simulink model "HQEV_MiL_20160830_integrate_r2017a"  (Simulink 8.9)
settings: Solver=FixedStepDiscrete  StartTime=0.0  StopTime=inf  FixedStep=0.01  RelTol=1e-3  EnableMultiTasking=on
PostLoadFcn:
  | , if any(exist('dsrtsu_mdlpostloadfcn', 'file') == [2, 3, 6]), try dsrtsu_mdlpostloadfcn('Execute', bdroot); catch fprintf('Error in PostLoadFcn (dsrtsu_mdlpostloadfcn) for model "%s":\n %s\n', bdroot, lasterr); end, end,
values from neighbouring files (symbols this model uses):
  Bat_C_Ah = 36    [parameter_V1.mat]
  Bat_ocv_xIndex = [5 10 20 30 40 50 60 70 80 90 95]    [parameter_V1.mat]
  Bat_ocv_z = [329 332 340 345 347 351 358 372 377 386 391]    [parameter_V1.mat]
  Bat_R_ohm_z = [4.41 3.46 1.57 1.07 0.76 0.63 0.55 0.44 0.41 0.4 0.4 3.14 ... (66 elements, 11x6)]    [parameter_V1.mat]
  Bat_SOC_Init = 90    [parameter_V1.mat]
  Env_hum_pct_Ambient = 30    [parameter_V1.mat]
  Env_Slope_deg = 0    [parameter_V1.mat]
  Env_Temp_degC_Ambient = 25    [parameter_V1.mat]
  Env_v_kmph_HWind = 0    [parameter_V1.mat]
  Reducer_F_i = 7.23    [parameter_V1.mat]
  Reducer_R_i = 7.23    [parameter_V1.mat]
  Veh =     [parameter_V1.mat]
  Veh_A_m2_Fr = 2.246    [parameter_V1.mat]
  Veh_F_Brake =     [parameter_V1.mat]
  Veh_fac_AirDrag = 0.326    [parameter_V1.mat]
  Veh_fac_WhDragFrict_0 = 0.011    [parameter_V1.mat]
  Veh_g_mps2_C = 9.81    [parameter_V1.mat]
  Veh_GainBrake =     [parameter_V1.mat]
  Veh_h_m_COGHigh = 0.5    [parameter_V1.mat]
  Veh_J_kgm2_Wh = 1.3635    [parameter_V1.mat]
  Veh_L_m_AxlBas = 2.63    [parameter_V1.mat]
  Veh_M_kg = 1427    [parameter_V1.mat]
  Veh_mu_Brake = 0.4    [parameter_V1.mat]
  Veh_mu_Tyre =     [parameter_V1.mat]
  Veh_num_FrictPair = 8    [parameter_V1.mat]
  Veh_pct_Brk = 70    [parameter_V1.mat]
  Veh_r_dyn =     [parameter_V1.mat]
  Veh_r_m_BrkDisk = 0.136    [parameter_V1.mat]
  Veh_rho_kgpm3_Air = 1.2258    [parameter_V1.mat]
undefined symbols (not defined in the file or in its folder): DiscIntNeverNeededParam, p_bool_False_M, p_bool_True_M
libraries: BaseOperationLib_Browser x38, simulink x8, DTQC_lib x1, ERR_lib x1, MQM_lib x1, PTCL_lib x1, PUD_lib x1, TQD_lib x1, TQR_lib x1, VMM_lib x1, ACCA_lib x1, BBCA_lib x1
(part 9 of 15)

== system HQEV_MiL_20160830_integrate_r2017a/MiL/Test_Integration/MCU_RR/MCU/Signal/MCU2_TMSpeed ==
  In1 : Inport
  Bus Selector : BusSelector  OutputSignals=signal1.Motor_R.EM2_spd
  out : Outport
  wires:
  In1/1 -> Bus Selector/1
  Bus Selector/1 -> out/1  "<EM2_spd>"

== system HQEV_MiL_20160830_integrate_r2017a/MiL/Test_Integration/MCU_RR/MCU/Signal/MCU2_TMStatus ==
  In1 : Inport
  Bus Selector : BusSelector  OutputSignals=signal2.MCU2_TMStatus
  out : Outport
  wires:
  In1/1 -> Bus Selector/1
  Bus Selector/1 -> out/1  "<MCU2_TMStatus>"

== system HQEV_MiL_20160830_integrate_r2017a/MiL/Test_Integration/MCU_RR/MCU/Signal/MCU2_TM_MAGTorque ==
  In1 : Inport
  Bus Selector : BusSelector  OutputSignals=signal2.MCU2_TMMAGTorque
  out : Outport
  wires:
  In1/1 -> Bus Selector/1
  Bus Selector/1 -> out/1  "<MCU2_TMMAGTorque>"

== system HQEV_MiL_20160830_integrate_r2017a/MiL/Test_Integration/MCU_RR/MCU/Signal/MCU2_TM_MAMTorque ==
  In1 : Inport
  Bus Selector : BusSelector  OutputSignals=signal2.MCU2_TMMAMTorque
  out : Outport
  wires:
  In1/1 -> Bus Selector/1
  Bus Selector/1 -> out/1  "<MCU2_TMMAMTorque>"

== system HQEV_MiL_20160830_integrate_r2017a/MiL/Test_Integration/MCU_RR/MCU/Signal/MCU2_trq_req ==
  In1 : Inport
  Bus Selector : BusSelector  OutputSignals=signal2.EM2_trq_Req
  out : Outport
  wires:
  In1/1 -> Bus Selector/1
  Bus Selector/1 -> out/1  "<EM2_trq_Req>"

== system HQEV_MiL_20160830_integrate_r2017a/MiL/Test_Integration/MCU_RR/MCU/Signal/MCU2_trq_req1 ==
  In1 : Inport
  Bus Selector : BusSelector  OutputSignals=signal2.MCUShutdownEnable
  out : Outport
  wires:
  Bus Selector/1 -> out/1  "<MCUShutdownEnable>"
  In1/1 -> Bus Selector/1

== system HQEV_MiL_20160830_integrate_r2017a/MiL/Test_Integration/Motor_FF/Motor/Motor/Uc_Management ==
  note: Uc+RC(dUc/dt)=Uterm
  MainPos_Contactor : Inport
  PreCharg_Contactor : Inport  Port=2
  MainNeg_Contactor : Inport  Port=3
  RapidDischargeEnable : Inport  Port=4
  Battery_Voltage : Inport  Port=5
  BMS_ChargePlusContactorCoilState : Inport  Port=6
  BMS_ChargeMinusContactorCoilState : Inport  Port=7
  Charger_Status : Inport  Port=8
  Bus Selector : BusSelector  OutputSignals=U_Term,RC
  Discrete-Time Integrator : DiscreteIntegrator  SampleTime=-1  ICPrevOutput=DiscIntNeverNeededParam  ICPrevScaledInput=DiscIntNeverNeededParam
  Divide : Product  Inputs=*/
  Multiport Switch : MultiPortSwitch  DataPortOrder=Zero-based contiguous  zeroidx=on
  Open : Subsystem
  PreCharg : Subsystem
  RelayLogic : Subsystem
  ShortCircle : Subsystem
  Subtract : Sum  Inputs=-+
  Uc : Outport
  wires:
  Subtract/1 -> Divide/1
  Divide/1 -> Discrete-Time Integrator/1
  Discrete-Time Integrator/1 -> Uc/1, Subtract/1, Open/2(Uc)
  PreCharg/1(Out) -> Multiport Switch/4
  ShortCircle/1(Out1) -> Multiport Switch/3
  Open/1(Out1) -> Multiport Switch/2
  Multiport Switch/1 -> Bus Selector/1
  Bus Selector/1 -> Subtract/2  "<U_Term>"
  Bus Selector/2 -> Divide/2  "<RC>"
  RapidDischargeEnable/1 -> Open/1(RapidDischargeEnable)
  Battery_Voltage/1 -> ShortCircle/1(Bat_U), PreCharg/1(Bat_U)
  MainPos_Contactor/1 -> RelayLogic/1(Main_Pos)
  PreCharg_Contactor/1 -> RelayLogic/2(PreCharg)
  MainNeg_Contactor/1 -> RelayLogic/3(Main_Neg)
  BMS_ChargePlusContactorCoilState/1 -> RelayLogic/4(ChargePos)
  BMS_ChargeMinusContactorCoilState/1 -> RelayLogic/5(ChargeNeg)
  Charger_Status/1 -> RelayLogic/6(Charger_Status)
  RelayLogic/1(Out1) -> Multiport Switch/1

== system HQEV_MiL_20160830_integrate_r2017a/MiL/Test_Integration/Motor_FF/Motor/Motor/eMotor ==
  n_FD_in : Inport
  T_req : Inport  Port=2
  Electric Power : Subsystem
  Motor Torque : Subsystem
  motor inertia : Constant  Value=0.08
  n_Motor : Outport
  P_Motor_elec : Outport  Port=2
  EM_trq : Outport  Port=3
  "J_out " : Outport  Port=4
  P_Motor_loss : Outport  Port=5
  wires:
  motor inertia/1 -> "J_out "/1
  Electric Power/1(P_Motor_elec) -> P_Motor_elec/1
  n_FD_in/1 -> Electric Power/1(n_Motor), n_Motor/1
  T_req/1 -> Motor Torque/1(MCU1_trq_req)
  Motor Torque/1(T_Motor) -> EM_trq/1, Electric Power/2(T_Motor)
  Electric Power/2(P_Motor_loss) -> P_Motor_loss/1

== system HQEV_MiL_20160830_integrate_r2017a/MiL/Test_Integration/Motor_RR/Motor/Motor1/Uc_Management ==
  note: Uc+RC(dUc/dt)=Uterm
  MainPos_Contactor : Inport
  PreCharg_Contactor : Inport  Port=2
  MainNeg_Contactor : Inport  Port=3
  RapidDischargeEnable : Inport  Port=4
  Battery_Voltage : Inport  Port=5
  BMS_ChargePlusContactorCoilState : Inport  Port=6
  BMS_ChargeMinusContactorCoilState : Inport  Port=7
  Charger_Status : Inport  Port=8
  Bus Selector : BusSelector  OutputSignals=U_Term,RC
  Discrete-Time Integrator : DiscreteIntegrator  SampleTime=-1  ICPrevOutput=DiscIntNeverNeededParam  ICPrevScaledInput=DiscIntNeverNeededParam
  Divide : Product  Inputs=*/
  Multiport Switch : MultiPortSwitch  DataPortOrder=Zero-based contiguous  zeroidx=on
  Open : Subsystem
  PreCharg : Subsystem
  RelayLogic : Subsystem
  ShortCircle : Subsystem
  Subtract : Sum  Inputs=-+
  Uc : Outport
  wires:
  Subtract/1 -> Divide/1
  Divide/1 -> Discrete-Time Integrator/1
  Discrete-Time Integrator/1 -> Uc/1, Subtract/1, Open/2(Uc)
  PreCharg/1(Out) -> Multiport Switch/4
  ShortCircle/1(Out1) -> Multiport Switch/3
  Open/1(Out1) -> Multiport Switch/2
  Multiport Switch/1 -> Bus Selector/1
  Bus Selector/1 -> Subtract/2  "<U_Term>"
  Bus Selector/2 -> Divide/2  "<RC>"
  RapidDischargeEnable/1 -> Open/1(RapidDischargeEnable)
  Battery_Voltage/1 -> ShortCircle/1(Bat_U), PreCharg/1(Bat_U)
  MainPos_Contactor/1 -> RelayLogic/1(Main_Pos)
  PreCharg_Contactor/1 -> RelayLogic/2(PreCharg)
  MainNeg_Contactor/1 -> RelayLogic/3(Main_Neg)
  BMS_ChargePlusContactorCoilState/1 -> RelayLogic/4(ChargePos)
  BMS_ChargeMinusContactorCoilState/1 -> RelayLogic/5(ChargeNeg)
  Charger_Status/1 -> RelayLogic/6(Charger_Status)
  RelayLogic/1(Out1) -> Multiport Switch/1

== system HQEV_MiL_20160830_integrate_r2017a/MiL/Test_Integration/Motor_RR/Motor/Motor1/eMotor ==
  n_FD_in : Inport
  T_req : Inport  Port=2
  Electric Power : Subsystem
  Motor Torque : Subsystem
  motor inertia : Constant  Value=0.08
  n_Motor : Outport
  P_Motor_elec : Outport  Port=2
  EM_trq : Outport  Port=3
  "J_out " : Outport  Port=4
  P_Motor_loss : Outport  Port=5
  wires:
  motor inertia/1 -> "J_out "/1
  Electric Power/1(P_Motor_elec) -> P_Motor_elec/1
  n_FD_in/1 -> Electric Power/1(n_Motor), n_Motor/1
  T_req/1 -> Motor Torque/1(MCU1_trq_req)
  Motor Torque/1(T_Motor) -> EM_trq/1, Electric Power/2(T_Motor)
  Electric Power/2(P_Motor_loss) -> P_Motor_loss/1

== system HQEV_MiL_20160830_integrate_r2017a/MiL/Test_Integration/Reducer_F/FinalDrive/FinalDrive/CalcJ_Ratio ==
  J_pre [kg*m^2] : Inport
  J_in : Constant  Value=0.01
  J_out : Constant  Value=0.01
  Math Function : Math  Operator=square  SaturateOnIntegerOverflow=on
  Product : Product  SaturateOnIntegerOverflow=on  OutDataTypeStr=Inherit: Same as first input
  Sum : Sum  Inputs=|++  SaturateOnIntegerOverflow=on
  Sum1 : Sum  Inputs=|++  SaturateOnIntegerOverflow=on
  ratio : Constant  Value=Reducer_F_i
  J_out [kg*m^2] : Outport
  wires:
  Sum1/1 -> J_out [kg*m^2]/1
  J_out/1 -> Sum1/2
  Product/1 -> Sum1/1
  Math Function/1 -> Product/2
  Sum/1 -> Product/1
  ratio/1 -> Math Function/1
  J_in/1 -> Sum/2
  J_pre [kg*m^2]/1 -> Sum/1

== system HQEV_MiL_20160830_integrate_r2017a/MiL/Test_Integration/Reducer_F/FinalDrive/FinalDrive/Subsystem ==
  T_in : Inport  Description=Input torque [Nm]
  n_Wheel : Inport  Description=Output speed of final drive [rad/s]  Port=2
  Backward : Subsystem
  Derection : Subsystem
  Forward : Subsystem
  Switch : Switch  Criteria=u2 > Threshold
  T_out : Outport
  wires:
  Derection/1(derection) -> Switch/2
  Forward/1(T_out) -> Switch/1
  Backward/1(T_out) -> Switch/3
  n_Wheel/1 -> Derection/1(n_Wheel)
  T_in/1 -> Backward/1(T_in), Derection/2(T_in), Forward/1(T_in)
  Switch/1 -> T_out/1

== system HQEV_MiL_20160830_integrate_r2017a/MiL/Test_Integration/Reducer_R/FinalDrive/FinalDrive/CalcJ_Ratio ==
  J_pre [kg*m^2] : Inport
  Constant : Constant  Value=0.01
  Constant1 : Constant  Value=0.01
  Constant2 : Constant  Value=Reducer_R_i
  Math Function : Math  Operator=square  SaturateOnIntegerOverflow=on
  Product : Product  SaturateOnIntegerOverflow=on  OutDataTypeStr=Inherit: Same as first input
  Sum : Sum  Inputs=|++  SaturateOnIntegerOverflow=on
  Sum1 : Sum  Inputs=|++  SaturateOnIntegerOverflow=on
  J_out [kg*m^2] : Outport
  wires:
  J_pre [kg*m^2]/1 -> Sum/1
  Constant/1 -> Sum/2
  Constant2/1 -> Math Function/1
  Sum/1 -> Product/1
  Math Function/1 -> Product/2
  Product/1 -> Sum1/1
  Constant1/1 -> Sum1/2
  Sum1/1 -> J_out [kg*m^2]/1

== system HQEV_MiL_20160830_integrate_r2017a/MiL/Test_Integration/Reducer_R/FinalDrive/FinalDrive/Subsystem ==
  T_in : Inport  Description=Input torque [Nm]
  n_Wheel : Inport  Description=Output speed of final drive [rad/s]  Port=2
  Backward : Subsystem
  Derection : Subsystem
  Forward : Subsystem
  Switch : Switch  Criteria=u2 ~= 0
  T_out : Outport
  wires:
  Switch/1 -> T_out/1
  T_in/1 -> Derection/2(T_in), Backward/1(T_in), Forward/1(T_in)
  n_Wheel/1 -> Derection/1(n_Wheel)
  Backward/1(T_out) -> Switch/3
  Forward/1(T_out) -> Switch/1
  Derection/1(derection) -> Switch/2

== system HQEV_MiL_20160830_integrate_r2017a/MiL/Test_Integration/Thermal/Thermal/Subsystem/Battery_Cooling_Circle ==
  PWM_BatteryPump : Inport
  AC_OnOff : Inport  Port=2
  PWM_PTC : Inport  Port=3
  pwr_BatteryLoss : Inport  Port=4
  BatTempIndex : Inport  Port=5
  Battery : Subsystem
  Chiller : Subsystem
  PTC : Subsystem
  Pump_Battery : Subsystem
  Scope : Scope
  Terminator1 : Terminator
  Terminator2 : Terminator
  Unit Delay1 : UnitDelay  SampleTime=-1
  Battery_Temp : Outport
  wires:
  AC_OnOff/1 -> Chiller/3(AC_OnOff)
  Chiller/3(NULL) -> Terminator1/1
  PTC/1(Q_water_outlet) -> Battery/1(T_water_Inlet)
  Pump_Battery/1(Q_Water_outlet) -> Chiller/1(Q_water_inlet)
  Pump_Battery/2(T_Water_outlet) -> Chiller/2(T_water_inlet)
  PWM_BatteryPump/1 -> Pump_Battery/1(PWM_Battery)
  Chiller/1(Q_water_outlet) -> PTC/1(Q_water_inlet)
  Chiller/2(T_water_outlet) -> PTC/2(T_water_inlet)
  PWM_PTC/1 -> PTC/3(PWM_PTC_pct)
  PTC/3(NULL) -> Terminator2/1
  Unit Delay1/1 -> Pump_Battery/2(T_Water_Inlet)
  PTC/2(T_water_outlet) -> Battery/2(Q_water_Inlet)
  pwr_BatteryLoss/1 -> Battery/3(pwr_BatteryLoss)
  Battery/1(T_Battery) -> Battery_Temp/1
  Battery/2(T_water_outlet) -> Unit Delay1/1
  BatTempIndex/1 -> Battery/4(BatTempIndex), Scope/1

== system HQEV_MiL_20160830_integrate_r2017a/MiL/Test_Integration/Thermal/Thermal/Subsystem/Motor_Cooling_Circle ==
  PWM_Pump1 : Inport
  pwr_Motor1Loss : Inport  Port=2
  PWM_Pump2 : Inport  Port=3
  pwr_Motor2Loss : Inport  Port=4
  PWM_Fan : Inport  Port=5
  pwr_ChargerLoss : Inport  Port=6
  pwr_DCDCLoss : Inport  Port=7
  Charger : Subsystem
  DCDC : Subsystem
  Motor_F : Subsystem
  Motor_R : Subsystem
  Multiple_Input_Joint : Subsystem
  Pump_F : Subsystem
  Pump_R : Subsystem
  Radiator : Subsystem
  Terminator1 : Terminator
  Unit Delay : UnitDelay  InitialCondition=25  SampleTime=-1
  Motor_F_Temp : Outport
  Motor_R_Temp : Outport  Port=2
  DCDC_Temp : Outport  Port=3
  Charger_Temp : Outport  Port=4
  wires:
  Motor_F/2(Q_water_outlet) -> Multiple_Input_Joint/1(Q1)
  Motor_F/3(T_water_outlet) -> Multiple_Input_Joint/2(T1)
  Pump_F/1(T_Water_outlet) -> Motor_F/1(T_water_Inlet)
  Pump_F/2(Q_Water_outlet) -> Motor_F/2(Q_water_Inlet)
  Pump_R/1(T_Water_outlet) -> Motor_R/1(T_water_Inlet)
  Multiple_Input_Joint/1(Q0) -> Radiator/1(Q_water_inlet)
  Multiple_Input_Joint/2(T0) -> Radiator/2(T_water_inlet)
  Radiator/3(NULL) -> Terminator1/1
  Motor_F/1(T_Motor) -> Motor_F_Temp/1
  PWM_Pump1/1 -> Pump_F/2(PWM_Pump1)
  PWM_Pump2/1 -> Pump_R/2(PWM_Pump2)
  pwr_Motor1Loss/1 -> Motor_F/3(pwr_MotorLoss)
  PWM_Fan/1 -> Radiator/3(PWM_Fan)
  Unit Delay/1 -> Pump_F/1(T_Water_Inlet), Pump_R/1(T_Water_Inlet)
  Pump_R/2(Q_Water_outlet) -> Motor_R/2(Q_water_Inlet)
  pwr_Motor2Loss/1 -> Motor_R/3(pwr_MotorLoss)
  Motor_R/1(Q_water_outlet) -> Multiple_Input_Joint/3(Q2)
  Motor_R/2(T_water_outlet) -> Multiple_Input_Joint/4(T2)
  Motor_R/3(T_Motor) -> Motor_R_Temp/1
  DCDC/1(T_DCDC) -> DCDC_Temp/1
  Radiator/1(Q_water_outlet) -> Charger/1(Q_water_Inlet)
  Radiator/2(T_water_outlet) -> Charger/2(T_water_Inlet)
  pwr_ChargerLoss/1 -> Charger/3(pwr_ChargerLoss)
  pwr_DCDCLoss/1 -> DCDC/3(pwr_DCDCLoss)
  Charger/1(T_Charger) -> DCDC/1(T_water_Inlet)
  Charger/3(T_water_outlet) -> Charger_Temp/1
  Charger/2(Q_water_outlet) -> DCDC/2(Q_water_Inlet)
  DCDC/2(T_water_outlet) -> Unit Delay/1

== system HQEV_MiL_20160830_integrate_r2017a/MiL/Test_Integration/Vehicle/Vehicle/Vehicle/J_Equivalent  ==
  J_in : Inport
  m_add [kg] : Inport  Description=Additional vehicle mass which kight be delivered by other components [kg]  Port=2
  Constant : Constant  Value=Veh_J_kgm2_Wh*4
  Constant1 : Constant  Value=Veh_M_kg
  Sum : Sum  SaturateOnIntegerOverflow=on
  Sum1 : Sum  Inputs=+++
  r_dyn^2 : Gain  Gain=Veh_r_dyn.z^2  SaturateOnIntegerOverflow=on  OutDataTypeStr=Inherit: Same as input  ParamDataTypeStr=Inherit: Same as input
  J_Equ : Outport
  m_total : Outport  Port=2
  wires:
  r_dyn^2/1 -> Sum1/1
  Constant/1 -> Sum1/2
  Sum1/1 -> J_Equ/1
  J_in/1 -> Sum1/3
  Constant1/1 -> Sum/1
  m_add [kg]/1 -> Sum/2
  Sum/1 -> m_total/1, r_dyn^2/1

== system HQEV_MiL_20160830_integrate_r2017a/MiL/Test_Integration/Vehicle/Vehicle/Vehicle/Resistance Torque ==
  v_Hwind [m/s] : Inport
  v_Veh [km/h] : Inport  Port=2
  phi_Slope [deg] : Inport  Port=3
  m_total [kg] : Inport  Port=4
  "  " : Product  SaturateOnIntegerOverflow=on  InputSameDT=on  OutDataTypeStr=Inherit: Same as first input
  " 1" : Gain  Gain=-1  SaturateOnIntegerOverflow=on  OutDataTypeStr=Inherit: Same as input  ParamDataTypeStr=Inherit: Same as input
  Constant1 : Constant
  Constant2 : Constant  Value=-1
  Sigmoid-Function : Subsystem  mask(VeLoDyn Basic Function){Offset=0, Damping=-100}
      mask help: Komplementaere Gewichtung der Eingaenge [x1*w und x2*(1-w)] gesteuert ueber Ctrl-Eingang.
      mask Help:
      | Sigmoid Funktion
      | Komplementaere Gewichtung der Eingaenge [x1*w und x2*(1-w)] gesteuert ueber
      | Ctrl-Eingang.
      | Offset und Steilheit der UEbergangsfunktion kann mit Parameter Offset und Daempfung
      | eingestellt werden.
      mask Display: plot([0:.01:10],(1./(1+exp(([0:.01:10]-5)*Damping))))
  Sum : Sum  SaturateOnIntegerOverflow=on  InputSameDT=on  OutDataTypeStr=Inherit: Same as first input
  Sum1 : Sum  SaturateOnIntegerOverflow=on  InputSameDT=on  OutDataTypeStr=Inherit: Same as first input
  Vehicle_r_dyn : Gain  Gain=Veh_r_dyn.z  SaturateOnIntegerOverflow=on  OutDataTypeStr=Inherit: Same as input  ParamDataTypeStr=Inherit: Same as input
  air_drag : Subsystem
  "km/h -> m/s" : Gain  Gain=1/3.6  SaturateOnIntegerOverflow=on  OutDataTypeStr=Inherit: Same as input  ParamDataTypeStr=Inherit: Same as input
  slope_drag : Subsystem
  wheel_drag : Subsystem
  T_Drag [Nm] : Outport
  wires:
  m_total [kg]/1 -> wheel_drag/2(m [kg]), slope_drag/1(m [kg])
  Vehicle_r_dyn/1 -> T_Drag [Nm]/1
  v_Veh [km/h]/1 -> air_drag/1(v_Veh [km/h]), "km/h -> m/s"/1, Sigmoid-Function/2(Ctrl)
  phi_Slope [deg]/1 -> wheel_drag/1(phi_Slope [deg]), slope_drag/2(phi_Slope [deg])
  air_drag/1(F_AirDrag [N]) -> Sum/2
  Sum/1 -> "  "/1
  "  "/1 -> Sum1/2
  slope_drag/1(F_Slope [N]) -> Sum1/1
  wheel_drag/1(" F_Wh_drag [N]") -> Sum/1
  Sigmoid-Function/1(y) -> " 1"/1
  v_Hwind [m/s]/1 -> air_drag/2(v_Hwind [m/s])
  Sum1/1 -> Vehicle_r_dyn/1
  " 1"/1 -> "  "/2
  Constant1/1 -> Sigmoid-Function/1(x1)
  Constant2/1 -> Sigmoid-Function/3(x2)
  "km/h -> m/s"/1 -> wheel_drag/3(v_Veh [m/s])

== system HQEV_MiL_20160830_integrate_r2017a/MiL/Test_Integration/Vehicle/Vehicle/Vehicle/Wheel Torque ==
  T_inFront [Nm] : Inport  Description=Input torque [Nm]
  T_inRear [Nm] : Inport  Description=Input torque [Nm]  Port=2
  Sig_Brake [%] : Inport  Description=Brake Signal of the driver [%]  Port=3
  phi_Slope [deg] : Inport  Port=4
  acc_Veh : Inport  Port=5
  m_total : Inport  Port=6
  Omega_wh : Inport  Description=Brake Signal of the driver [%]  Port=7
  Brake : Subsystem
  Wheel_Torque : Subsystem
  maximal_wheel_torque : Subsystem
  T_wheel : Outport
  wires:
  Brake/1(T_Brake [Nm]) -> Wheel_Torque/5(T_Brake [Nm])
  T_inFront [Nm]/1 -> Wheel_Torque/3(T_inFront [Nm])
  maximal_wheel_torque/1(T_maxFront [Nm]) -> Wheel_Torque/1(T_maxFront [Nm])
  Wheel_Torque/1(T_Wheel_lim [Nm]) -> T_wheel/1
  acc_Veh/1 -> maximal_wheel_torque/2(acc_Vehicle [m/s^2])
  maximal_wheel_torque/2(T_maxRear [Nm]) -> Wheel_Torque/2(T_maxRear [Nm])
  Sig_Brake [%]/1 -> Brake/1(Sig_Brake [%])
  m_total/1 -> maximal_wheel_torque/3(m [kg])
  T_inRear [Nm]/1 -> Wheel_Torque/4(T_inRear [Nm])
  phi_Slope [deg]/1 -> maximal_wheel_torque/1(phi_Slope [deg])
  Omega_wh/1 -> Brake/2(Omega_wh [rad/s])

== system HQEV_MiL_20160830_integrate_r2017a/MiL/Test_Integration/Vehicle/Vehicle/Vehicle/dw_Correction ==
  dOmega_out : Inport
  "Omega_out " : Inport  Port=2
  1/r_dyn.1 : Gain  Gain=1/1000  SaturateOnIntegerOverflow=on  OutDataTypeStr=Inherit: Same as input  ParamDataTypeStr=Inherit: Same as input
  1/r_dyn.2 : Gain  Gain=3.6  SaturateOnIntegerOverflow=on  OutDataTypeStr=Inherit: Same as input  ParamDataTypeStr=Inherit: Same as input
  1/r_dyn.3 : Gain  Gain=30/pi  SaturateOnIntegerOverflow=on  OutDataTypeStr=Inherit: Same as input  ParamDataTypeStr=Inherit: Same as input
  Constant2 : Constant  Value=0
  Discrete-Time Integrator : DiscreteIntegrator  SampleTime=-1  ICPrevOutput=DiscIntNeverNeededParam  ICPrevScaledInput=DiscIntNeverNeededParam
  Relational Operator : RelationalOperator  Operator=~=  RndMeth=Nearest
  Switch : Switch  Threshold=0.5  SaturateOnIntegerOverflow=on
  Unit Delay : UnitDelay  SampleTime=-1
  Unit Delay1 : UnitDelay  SampleTime=-1
  r_Dyn : Gain  Gain=Veh_r_dyn.z  SaturateOnIntegerOverflow=on  OutDataTypeStr=Inherit: Same as input  ParamDataTypeStr=Inherit: Same as input
  r_Dyn1 : Gain  Gain=Veh_r_dyn.z  SaturateOnIntegerOverflow=on  OutDataTypeStr=Inherit: Same as input  ParamDataTypeStr=Inherit: Same as input
  dist [km] : Outport
  n_Wh : Outport  Port=2
  v_Veh [km/h] : Outport  Port=3
  acc [m/s^2] : Outport  Port=4
  wires:
  r_Dyn/1 -> Unit Delay1/1
  Unit Delay/1 -> Relational Operator/1
  Relational Operator/1 -> Switch/2
  Constant2/1 -> Switch/3
  dOmega_out/1 -> Switch/1
  "Omega_out "/1 -> Relational Operator/2, Unit Delay/1, r_Dyn1/1, 1/r_dyn.3/1
  Switch/1 -> r_Dyn/1
  1/r_dyn.1/1 -> Discrete-Time Integrator/1
  Discrete-Time Integrator/1 -> dist [km]/1
  1/r_dyn.2/1 -> v_Veh [km/h]/1
  r_Dyn1/1 -> 1/r_dyn.1/1, 1/r_dyn.2/1
  Unit Delay1/1 -> acc [m/s^2]/1
  1/r_dyn.3/1 -> n_Wh/1

== system HQEV_MiL_20160830_integrate_r2017a/MiL/Test_Integration/BMS/BMS/BMS/BMS/Charge_Control ==
  CC : Inport
  CC2 : Inport  Port=2
  SOC : Inport  Port=3
  Bat_temp : Inport  Port=4
  HCU_ChargePermission : Inport  Port=5
  HCU_ChargeHeatingPermission : Inport  Port=6
  BMS_HeatingRequest : Inport  Port=7
  BMS_InsulationMonitorWarningIN : Inport  Port=8
  AC Charge connect : Subsystem
  Bus Creator : BusCreator  Inputs=10
  Bus Creator1 : BusCreator  Inputs=10
  Bus Creator2 : BusCreator  Inputs=10
  Bus Selector : BusSelector  OutputSignals=signal1,signal2,signal3,signal4,signal5,signal6,signal7,signal8,signal9,signal10
  Connection_Check : Subsystem
  Constant : Constant  Value=0
  Constant1 : Constant  Value=2
  DC Charge connect : Subsystem
  Disconnect : Subsystem
  Multiport Switch : MultiPortSwitch  DataPortOrder=Zero-based contiguous  zeroidx=on
  Switch1 : Switch  Criteria=u2 ~= 0  OutDataTypeStr=uint8
  Switch2 : Switch  Criteria=u2 ~= 0  OutDataTypeStr=uint8
  BMS ChargeRequest : Outport
  BMS_ChargeStationOutputCurrent : Outport  Port=2
  BMS_ChargeStationOutputVoltage : Outport  Port=3
  BMS_InstantPowerConsumption : Outport  Port=4
  BMS_ChargeStationParameterConfigStatus : Outport  Port=5
  BMS_ChargeStationStatus : Outport  Port=6
  BMS_RemainingChargeTime : Outport  Port=7
  BMS_InsulationMonitorWarning : Outport  Port=8
  BMS_ChargeStationHandShakeStatus : Outport  Port=9
  BMS_ChargeStatus : Outport  Port=10
  wires:
  Connection_Check/1(Out1) -> Multiport Switch/1
  Disconnect/1(BMS ChargeRequest) -> Bus Creator/1
  Disconnect/2(BMS_ChargeStationOutputCurrent) -> Bus Creator/2
  Disconnect/3(BMS_ChargeStationOutputVoltage) -> Bus Creator/3
  Disconnect/4(BMS_InstantPowerConsumption) -> Bus Creator/4
  Disconnect/5(BMS_ChargeStationParameterConfigStatus) -> Bus Creator/5
  Disconnect/6(BMS_ChargeStationStatus) -> Bus Creator/6
  Disconnect/7(BMS_RemainingChargeTime) -> Bus Creator/7
  Disconnect/8(BMS_InsulationMonitorWarning) -> Bus Creator/8
  Disconnect/9(BMS_ChargeStationHandShakeStatus) -> Bus Creator/9
  DC Charge connect/1(BMS ChargeRequest) -> Bus Creator1/1
  DC Charge connect/2(BMS_ChargeStationOutputCurrent) -> Bus Creator1/2
  DC Charge connect/3(BMS_ChargeStationOutputVoltage) -> Bus Creator1/3
  DC Charge connect/4(BMS_InstantPowerConsumption) -> Bus Creator1/4
  DC Charge connect/5(BMS_ChargeStationParameterConfigStatus) -> Bus Creator1/5
  DC Charge connect/6(BMS_ChargeStationStatus) -> Bus Creator1/6
  DC Charge connect/7(BMS_RemainingChargeTime) -> Bus Creator1/7
  DC Charge connect/8(BMS_InsulationMonitorWarning) -> Bus Creator1/8
  DC Charge connect/9(BMS_ChargeStationHandShakeStatus) -> Bus Creator1/9
  AC Charge connect/1(BMS ChargeRequest) -> Bus Creator2/1
  AC Charge connect/2(BMS_ChargeStationOutputCurrent) -> Bus Creator2/2
  AC Charge connect/3(BMS_ChargeStationOutputVoltage) -> Bus Creator2/3
  AC Charge connect/4(BMS_InstantPowerConsumption) -> Bus Creator2/4
  AC Charge connect/5(BMS_ChargeStationParameterConfigStatus) -> Bus Creator2/5
  AC Charge connect/6(BMS_ChargeStationStatus) -> Bus Creator2/6
  AC Charge connect/7(BMS_RemainingChargeTime) -> Bus Creator2/7
  AC Charge connect/8(BMS_InsulationMonitorWarning) -> Bus Creator2/8
  AC Charge connect/9(BMS_ChargeStationHandShakeStatus) -> Bus Creator2/9
  Bus Creator/1 -> Multiport Switch/2
  Bus Creator1/1 -> Multiport Switch/3
  Bus Creator2/1 -> Multiport Switch/4
  Multiport Switch/1 -> Bus Selector/1
  Bus Selector/2 -> BMS_ChargeStationOutputCurrent/1  "<signal2>"
  Bus Selector/3 -> BMS_ChargeStationOutputVoltage/1  "<signal3>"
  Bus Selector/4 -> BMS_InstantPowerConsumption/1  "<signal4>"
  Bus Selector/5 -> BMS_ChargeStationParameterConfigStatus/1  "<signal5>"
  Bus Selector/6 -> BMS_ChargeStationStatus/1  "<signal6>"
  Bus Selector/7 -> BMS_RemainingChargeTime/1  "<signal7>"
  Bus Selector/9 -> BMS_ChargeStationHandShakeStatus/1  "<signal9>"
  CC/1 -> Connection_Check/1(CC)
  CC2/1 -> Connection_Check/2(CC2), DC Charge connect/1(CC2)
  SOC/1 -> DC Charge connect/2(SOC), AC Charge connect/1(SOC)
  Bat_temp/1 -> DC Charge connect/3(Bat_temp), AC Charge connect/2(Bat_temp)
  HCU_ChargePermission/1 -> AC Charge connect/3(HCU_ChargePermission), DC Charge connect/4(HCU_ChargePermission)
  Disconnect/10(BMS_ChargeStatus) -> Bus Creator/10
  DC Charge connect/10(BMS_ChargeStatus) -> Bus Creator1/10
  AC Charge connect/10(BMS_ChargeStatus) -> Bus Creator2/10
  Bus Selector/10 -> BMS_ChargeStatus/1  "<signal10>"
  HCU_ChargeHeatingPermission/1 -> AC Charge connect/4(HCU_ChargeHeatingPermission), DC Charge connect/5(HCU_ChargeHeatingPermission)
  BMS_HeatingRequest/1 -> Switch2/2
  Constant/1 -> Switch2/1
  Bus Selector/1 -> Switch2/3  "<signal1>"
  Switch2/1 -> BMS ChargeRequest/1
  BMS_InsulationMonitorWarningIN/1 -> Switch1/2
  Bus Selector/8 -> Switch1/3  "<signal8>"
  Switch1/1 -> BMS_InsulationMonitorWarning/1
  Constant1/1 -> Switch1/1

== system HQEV_MiL_20160830_integrate_r2017a/MiL/Test_Integration/BMS/BMS/BMS/BMS/Power_Limit ==
  Constant{,1..3} (4 alike) : Constant  Value=100
  BatteryChargePowerAvailable_10 : Outport
  BMS_BatteryDischargePowerAvailable_10 : Outport  Port=2
  BMS_BatteryChargePowerAvailable_2 : Outport  Port=3
  BMS_BatteryDischargePowerAvailable_2 : Outport  Port=4
  wires:
  Constant/1 -> BatteryChargePowerAvailable_10/1
  Constant1/1 -> BMS_BatteryDischargePowerAvailable_10/1
  Constant2/1 -> BMS_BatteryChargePowerAvailable_2/1
  Constant3/1 -> BMS_BatteryDischargePowerAvailable_2/1

== system HQEV_MiL_20160830_integrate_r2017a/MiL/Test_Integration/BMS/BMS/BMS/BMS/Relay_Control ==
  MainPosContactorCtrl : Inport
  MainNegContactorCtrl : Inport  Port=2
  PrechargContactorCtrl : Inport  Port=3
  ChargPosContactorCtrl : Inport  Port=4
  ChargNegContactorCtrl : Inport  Port=5
  Relay : Subsystem
  Relay1 : Subsystem
  Relay2 : Subsystem
  Relay3 : Subsystem
  Relay4 : Subsystem
  MainPosContactorState : Outport
  MainNegContactorCoilState : Outport  Port=2
  PrechargeContactorCoilState : Outport  Port=3
  ChargePlusContactorState : Outport  Port=4
  ChargNegContactorCoilState : Outport  Port=5
  wires:
  Relay/1(Out1) -> MainPosContactorState/1
  Relay1/1(Out1) -> MainNegContactorCoilState/1
  Relay2/1(Out1) -> PrechargeContactorCoilState/1
  Relay3/1(Out1) -> ChargePlusContactorState/1
  Relay4/1(Out1) -> ChargNegContactorCoilState/1
  MainPosContactorCtrl/1 -> Relay/1(In1)
  MainNegContactorCtrl/1 -> Relay1/1(In1)
  PrechargContactorCtrl/1 -> Relay2/1(In1)
  ChargPosContactorCtrl/1 -> Relay3/1(In1)
  ChargNegContactorCtrl/1 -> Relay4/1(In1)

== system HQEV_MiL_20160830_integrate_r2017a/MiL/Test_Integration/BMS/BMS/BMS/BMS/State_Control ==
  SOC : Inport
  SOH : Inport  Port=2
  BMS_SOH : Outport
  BMS_SOC : Outport  Port=2
  BMS_RemainingEnergyRatio : Outport  Port=3
  wires:
  SOH/1 -> BMS_SOH/1
  SOC/1 -> BMS_SOC/1, BMS_RemainingEnergyRatio/1

== system HQEV_MiL_20160830_integrate_r2017a/MiL/Test_Integration/BMS/BMS/BMS/BMS/Thermal_Manage ==
  Battery_Temp : Inport
  CC : Inport  Port=2
  CC2 : Inport  Port=3
  Constant1 : Constant  Value=0
  Constant2 : Constant  Value=3
  Constant3 : Constant  Value=0
  Constant5 : Constant  Value=-20
  Constant8 : Constant  Value=-17
  Relational Operator : RelationalOperator  Operator=<=  OutDataTypeStr=boolean  RndMeth=Nearest
  Relational Operator1 : RelationalOperator  Operator=>  OutDataTypeStr=boolean  RndMeth=Nearest
  Relational Operator2 : RelationalOperator  Operator=<  OutDataTypeStr=boolean  RndMeth=Nearest
  Relational Operator3 : RelationalOperator  Operator=>  OutDataTypeStr=boolean  RndMeth=Nearest
  S-R Flip-Flop : BaseOperationLib_Browser/Others Unchanged/S-R Flip-Flop  SystemSampleTime=-1  initial_condition=0
  S-R Flip-Flop1 : BaseOperationLib_Browser/Others Unchanged/S-R Flip-Flop  SystemSampleTime=-1  initial_condition=0
  Switch : Switch  Criteria=u2 > Threshold
  Switch1 : Switch  Criteria=u2 > Threshold
  Terminator : Terminator
  Terminator1 : Terminator
  Bat_temp_Max : Outport
  Bat_temp_Min : Outport  Port=2
  Bat_temp_ave : Outport  Port=3
  Bat_temp_water : Outport  Port=4
  BMS_HeatingRequest : Outport  Port=5
  wires:
  S-R Flip-Flop/2 -> Terminator/1
  Battery_Temp/1 -> Relational Operator/1, Bat_temp_water/1, Bat_temp_ave/1, Bat_temp_Min/1, Bat_temp_Max/1, Relational Operator1/1, Relational Operator2/1, Relational Operator3/1
  Constant5/1 -> Relational Operator/2
  Relational Operator/1 -> S-R Flip-Flop/1
  Constant8/1 -> Relational Operator1/2
  Relational Operator1/1 -> S-R Flip-Flop/2
  Constant1/1 -> Relational Operator2/2
  Constant2/1 -> Relational Operator3/2
  Relational Operator3/1 -> S-R Flip-Flop1/2
  Relational Operator2/1 -> S-R Flip-Flop1/1
  S-R Flip-Flop1/2 -> Terminator1/1
  Switch/1 -> BMS_HeatingRequest/1
  Constant3/1 -> Switch1/3
  CC2/1 -> Switch1/2
  S-R Flip-Flop1/1 -> Switch1/1
  Switch1/1 -> Switch/3
  CC/1 -> Switch/2
  S-R Flip-Flop/1 -> Switch/1

== system HQEV_MiL_20160830_integrate_r2017a/MiL/Test_Integration/Battery/Battery/Battery/Battery_Output/Battery_characteristic ==
  SOC : Inport
  Battery_Temp : Inport  Port=2
  Lookup Table (2-D) : Lookup2D  RowIndex=Bat_R_ohm_rowIndex  ColumnIndex=Bat_R_ohm_columnIndex  Table=Bat_R_ohm_z
  OCV_Subsystem : Lookup  InputValues=Bat_ocv_xIndex  Table=Bat_ocv_z
  OCV : Outport
  ohm : Outport  Port=2
  wires:
  SOC/1 -> OCV_Subsystem/1, Lookup Table (2-D)/1
  OCV_Subsystem/1 -> OCV/1
  Lookup Table (2-D)/1 -> ohm/1
  Battery_Temp/1 -> Lookup Table (2-D)/2

== system HQEV_MiL_20160830_integrate_r2017a/MiL/Test_Integration/Battery/Battery/Battery/Battery_Output/Subsystem ==
  OCV : Inport
  Internal_Resistance : Inport  Port=2
  Bat_pwr_out : Inport  Port=3
  Current : Subsystem
  I*I : Product  RndMeth=Zero
  I*I*R : Product  RndMeth=Zero
  I*R : Product  RndMeth=Zero
  Uout : Sum  Inputs=+-
  maxmin : Saturate  UpperLimit=500  LowerLimit=200
  Bat_Voltage : Outport
  Bat_Current : Outport  Port=2
  Bat_pwr_loss : Outport  Port=3
  wires:
  I*R/1 -> Uout/2
  Uout/1 -> maxmin/1
  maxmin/1 -> Bat_Voltage/1, Current/1(U_out)
  Bat_pwr_out/1 -> Current/2(Bat_pwr_out)
  OCV/1 -> Uout/1
  Internal_Resistance/1 -> I*R/1, I*I*R/2
  Current/1(Battery_Current) -> Bat_Current/1, I*R/2, I*I/2, I*I/1
  I*I/1 -> I*I*R/1
  I*I*R/1 -> Bat_pwr_loss/1

== system HQEV_MiL_20160830_integrate_r2017a/MiL/Test_Integration/Charger/Charger/Charger/Charger/Abnormal ==
  function : TriggerPort  TriggerType=function-call  VariantControl=Variant
  Bus Creator : BusCreator  Inputs=5
  Subsystem : Subsystem
  Out1 : Outport
  wires:
  Bus Creator/1 -> Out1/1
  Subsystem/1(ChargerOutputVoltage) -> Bus Creator/1  "ChargerOutputVoltage"
  Subsystem/2(ChargerOutputCurrent) -> Bus Creator/2  "ChargerOutputCurrent"
  Subsystem/3(ChargerStatus) -> Bus Creator/3  "ChargerStatus"
  Subsystem/4(RechargeRequest) -> Bus Creator/4  "RechargeRequest"
  Subsystem/5(ChargerTemperature) -> Bus Creator/5  "ChargerTemperature"

== system HQEV_MiL_20160830_integrate_r2017a/MiL/Test_Integration/Charger/Charger/Charger/Charger/Fault ==
  function : TriggerPort  TriggerType=function-call  VariantControl=Variant
  Bus Creator : BusCreator  Inputs=5
  Subsystem : Subsystem
  Out1 : Outport
  wires:
  Bus Creator/1 -> Out1/1
  Subsystem/1(ChargerOutputVoltage) -> Bus Creator/1  "ChargerOutputVoltage"
  Subsystem/2(ChargerOutputCurrent) -> Bus Creator/2  "ChargerOutputCurrent"
  Subsystem/3(ChargerStatus) -> Bus Creator/3  "ChargerStatus"
  Subsystem/4(RechargeRequest) -> Bus Creator/4  "RechargeRequest"
  Subsystem/5(ChargerTemperature) -> Bus Creator/5  "ChargerTemperature"

== system HQEV_MiL_20160830_integrate_r2017a/MiL/Test_Integration/Charger/Charger/Charger/Charger/Idle ==
  CC : Inport
  ACChargeStation_U : Inport  Port=2
  function : TriggerPort  TriggerType=function-call  VariantControl=Variant
  Bus Creator1 : BusCreator  Inputs=5
  Subsystem : Subsystem
  Out : Outport
  wires:
  CC/1 -> Subsystem/1(CC)
  ACChargeStation_U/1 -> Subsystem/2(ACChargeStation_U)
  Subsystem/1(ChargerOutputVoltage) -> Bus Creator1/1  "ChargerOutputVoltage"
  Subsystem/2(ChargerOutputCurrent) -> Bus Creator1/2  "ChargerOutputCurrent"
  Subsystem/3(ChargerStatus) -> Bus Creator1/3  "ChargerStatus"
  Subsystem/4(RechargeRequest) -> Bus Creator1/4  "RechargeRequest"
  Subsystem/5(ChargerTemperature) -> Bus Creator1/5  "ChargerTemperature"
  Bus Creator1/1 -> Out/1

== system HQEV_MiL_20160830_integrate_r2017a/MiL/Test_Integration/Charger/Charger/Charger/Charger/Work ==
  HCU_ChargePermission : Inport
  BMS_MainPosContactorState : Inport  Port=2
  HCU_ChargeHeatingPermission : Inport  Port=3
  BMS_MainNegContactorState : Inport  Port=4
  BMS_PreChargeContactorState : Inport  Port=5
  BMS_ChargePosContactorState : Inport  Port=6
  BMS_ChargeNegContactorState : Inport  Port=7
  function : TriggerPort  TriggerType=function-call  VariantControl=Variant
  Bus Creator : BusCreator  Inputs=5
  Subsystem : Subsystem
  Out1 : Outport
  wires:
  Bus Creator/1 -> Out1/1
  HCU_ChargePermission/1 -> Subsystem/1(HCU_ChargePermission)
  BMS_MainPosContactorState/1 -> Subsystem/2(BMS_MainPosContactorState)
  HCU_ChargeHeatingPermission/1 -> Subsystem/3(HCU_ChargeHeatingPermission)
  BMS_MainNegContactorState/1 -> Subsystem/4(BMS_MainNegContactorState)
  BMS_PreChargeContactorState/1 -> Subsystem/5(BMS_PreChargeContactorState)
  BMS_ChargePosContactorState/1 -> Subsystem/6(BMS_ChargePosContactorState)
  BMS_ChargeNegContactorState/1 -> Subsystem/7(BMS_ChargeNegContactorState)
  Subsystem/1(ChargerOutputVoltage) -> Bus Creator/1  "ChargerOutputVoltage"
  Subsystem/2(ChargerOutputCurrent) -> Bus Creator/2  "ChargerOutputCurrent"
  Subsystem/3(ChargerStatus) -> Bus Creator/3  "ChargerStatus"
  Subsystem/4(RechargeRequest) -> Bus Creator/4  "RechargeRequest"
  Subsystem/5(ChargerTemperature) -> Bus Creator/5  "ChargerTemperature"

== system HQEV_MiL_20160830_integrate_r2017a/MiL/Test_Integration/Charger/Charger/Charger/Charger/mode_transfer ==
  HCU_ChargePermission : Inport
  HCU_HeatPermission : Inport  Port=2
  Constant : Constant  Value=0
  Constant1 : Constant  Value=0
  Logical Operator : Logic  Operator=NOT  AllPortsSameDT=off  OutDataTypeStr=boolean
  Logical Operator1 : Logic  Operator=OR  AllPortsSameDT=off  OutDataTypeStr=boolean
  Charger_Fault : Outport
  Charge_Enable : Outport  Port=2
  Charge_Finish : Outport  Port=3
  Charger_Abnormal : Outport  Port=4
  wires:
  Constant/1 -> Charger_Fault/1
  Constant1/1 -> Charger_Abnormal/1
  HCU_ChargePermission/1 -> Logical Operator1/1
  Logical Operator/1 -> Charge_Finish/1
  HCU_HeatPermission/1 -> Logical Operator1/2
  Logical Operator1/1 -> Charge_Enable/1, Logical Operator/1

== system HQEV_MiL_20160830_integrate_r2017a/MiL/Test_Integration/DCDC/DCDC/DCDC/Electric_Manage/DCDCStatus ==
  DCDC_Enable : Inport
  IO_In1 : Inport  Port=2
  Bus Selector : BusSelector  OutputSignals=IO.DCDC_ErrorSet
  DCDC_ErrorSET : Constant
  DCDC_NormalError : Constant  Value=2
  DCDC_NotWorking : Constant  Value=0
  DCDC_Working : Constant
  Relational Operator1 : RelationalOperator  Operator===  OutDataTypeStr=boolean  RndMeth=Nearest
  Switch : Switch  Criteria=u2 ~= 0  Threshold=0.5
  Switch1 : Switch  Criteria=u2 ~= 0  Threshold=0.5
  Unit Delay : UnitDelay  SampleTime=-1
  StatusDCDC : Outport
  wires:
  Unit Delay/1 -> Switch/2
  DCDC_Working/1 -> Switch/1
  DCDC_NotWorking/1 -> Switch/3
  DCDC_Enable/1 -> Unit Delay/1
  DCDC_ErrorSET/1 -> Relational Operator1/2
  Relational Operator1/1 -> Switch1/2
  Bus Selector/1 -> Relational Operator1/1  "<DCDC_ErrorSet>"
  Switch/1 -> Switch1/3
  Switch1/1 -> StatusDCDC/1
  IO_In1/1 -> Bus Selector/1
  DCDC_NormalError/1 -> Switch1/1

== system HQEV_MiL_20160830_integrate_r2017a/MiL/Test_Integration/Driver/Driver/Driver_AutoPedal/CTRL AccPed/Brake off ==
  u : Inport
  Compare : RelationalOperator  Operator=<=  OutDataTypeStr=uint(8)  ZeroCross=off  RndMeth=Nearest  InputSameDT=on
  Constant : Constant  Value=const  OutDataTypeStr=Inherit: Inherit via back propagation
  y : Outport
  wires:
  u/1 -> Compare/1
  Constant/1 -> Compare/2
  Compare/1 -> y/1

== system HQEV_MiL_20160830_integrate_r2017a/MiL/Test_Integration/Driver/Driver/Driver_AutoPedal/CTRL AccPed/Reset ==
  v_error : Inport
  v_Set : Inport  Port=2
  Brake [%] : Inport  Port=3
  Compare To Constant : Subsystem  mask(Compare To Constant){relop=<, const=-10, LogicOutDataTypeMode=boolean, ZeroCross=off}
      mask prompts: relop "Operator:"; const "Constant value:"; LogicOutDataTypeMode "Output data type mode:"; ZeroCross "Enable zero crossing detection"
      mask help: Determine how a signal compares to a constant.
      mask init: same as HQEV_MiL_20160830_integrate_r2017a/MiL/Test_Integration/Driver/Driver/Driver_AutoPedal/CTRL AccPed/Brake off
      mask TypeOptions relop: == | ~= | < | <= | >= | >
      mask TypeOptions LogicOutDataTypeMode: uint8 | boolean
      mask Callback ZeroCross: sl('zeroCrossEnable', gcbh);
      mask Display: disp(str)
  Compare To Constant1 : Subsystem  mask(Compare To Constant){relop=>, const=1, LogicOutDataTypeMode=boolean, ZeroCross=off}
      mask prompts: relop "Operator:"; const "Constant value:"; LogicOutDataTypeMode "Output data type mode:"; ZeroCross "Enable zero crossing detection"
      mask help: Determine how a signal compares to a constant.
      mask init: same as HQEV_MiL_20160830_integrate_r2017a/MiL/Test_Integration/Driver/Driver/Driver_AutoPedal/CTRL AccPed/Brake off
      mask TypeOptions relop: == | ~= | < | <= | >= | >
      mask TypeOptions LogicOutDataTypeMode: uint8 | boolean
      mask Callback ZeroCross: sl('zeroCrossEnable', gcbh);
      mask Display: disp(str)
  Data Type Conversion : DataTypeConversion  OutDataTypeStr=boolean
  Data Type Conversion1 : DataTypeConversion  OutDataTypeStr=double
  Data Type Conversion2 : DataTypeConversion  OutDataTypeStr=double
  Data Type Conversion3 : DataTypeConversion  OutDataTypeStr=boolean
  Hit  Crossing : HitCross  HitCrossingOffset=0.5
  Hit  Crossing1 : HitCross  HitCrossingOffset=0.5
  Logical Operator : Logic  Operator=OR  Inputs=3  AllPortsSameDT=off  OutDataTypeStr=boolean
  "v_Set==0 " : Subsystem  mask(Compare To Constant){relop=<=, const=eps, LogicOutDataTypeMode=uint8, ZeroCross=off}
      mask prompts: relop "Operator:"; const "Constant value:"; LogicOutDataTypeMode "Output data type mode:"; ZeroCross "Enable zero crossing detection"
      mask help: Determine how a signal compares to a constant.
      mask init: same as HQEV_MiL_20160830_integrate_r2017a/MiL/Test_Integration/Driver/Driver/Driver_AutoPedal/CTRL AccPed/Brake off
      mask TypeOptions relop: == | ~= | < | <= | >= | >
      mask TypeOptions LogicOutDataTypeMode: uint8 | boolean
      mask Callback ZeroCross: sl('zeroCrossEnable', gcbh);
      mask Display: disp(str)
  reset : Outport
  wires:
  "v_Set==0 "/1(y) -> Data Type Conversion1/1
  Compare To Constant1/1(y) -> Data Type Conversion2/1
  Brake [%]/1 -> Compare To Constant1/1(u)
  Compare To Constant/1(y) -> Logical Operator/1
  Hit  Crossing/1 -> Data Type Conversion/1
  Data Type Conversion/1 -> Logical Operator/3
  Data Type Conversion1/1 -> Hit  Crossing/1
  Data Type Conversion2/1 -> Hit  Crossing1/1
  Hit  Crossing1/1 -> Data Type Conversion3/1
  Data Type Conversion3/1 -> Logical Operator/2
  v_error/1 -> Compare To Constant/1(u)
  Logical Operator/1 -> reset/1
  v_Set/1 -> "v_Set==0 "/1(u)

== system HQEV_MiL_20160830_integrate_r2017a/MiL/Test_Integration/Driver/Driver/Driver_AutoPedal/CTRL AccPed/Subsystem ==
  v_Set : Inport
  v_Veh : Inport  Port=2
  Sum2 : Sum  Inputs=|+-  SaturateOnIntegerOverflow=on  InputSameDT=on  OutDataTypeStr=Inherit: Same as first input
  error : Outport
  wires:
  Sum2/1 -> error/1
  v_Set/1 -> Sum2/1
  v_Veh/1 -> Sum2/2

== system HQEV_MiL_20160830_integrate_r2017a/MiL/Test_Integration/Driver/Driver/Driver_AutoPedal/CTRL BrakePed/PI-Regler ==
  error : Inport
  Enable : EnablePort  StatesWhenEnabling=reset
  Discrete-Time Integrator : DiscreteIntegrator  SampleTime=-1  LimitOutput=on  UpperSaturationLimit=50  LowerSaturationLimit=-20  ICPrevOutput=DiscIntNeverNeededParam  ICPrevScaledInput=DiscIntNeverNeededParam
  I_value : Gain  Gain=0.1  SaturateOnIntegerOverflow=on  OutDataTypeStr=Inherit: Same as input  ParamDataTypeStr=Inherit: Same as input
  P_value : Gain  Gain=0.1  SaturateOnIntegerOverflow=on  OutDataTypeStr=Inherit: Same as input  ParamDataTypeStr=Inherit: Same as input
  Saturation : Saturate  UpperLimit=100  LowerLimit=0
  Sum : Sum  Inputs=|++  SaturateOnIntegerOverflow=on  InputSameDT=on  OutDataTypeStr=Inherit: Same as first input
  Result : Outport  OutputWhenDisabled=reset  InitialOutput=0
  wires:
  I_value/1 -> Discrete-Time Integrator/1
  P_value/1 -> Sum/1  "P-Anteil"
  error/1 -> P_value/1, I_value/1
  Sum/1 -> Saturation/1  "result"
  Saturation/1 -> Result/1
  Discrete-Time Integrator/1 -> Sum/2  "I-Anteil"

== system HQEV_MiL_20160830_integrate_r2017a/MiL/Test_Integration/Driver/Driver/Driver_AutoPedal/CTRL BrakePed/Reset_Block ==
  delta_v_set : Inport
  v_error : Inport  Port=2
  v_Veh : Inport  Port=3
  Brake : Inport  Port=4
  Brake_Set : Inport  Port=5
  Compare To Constant2 : Subsystem  mask(Compare To Constant){relop=>, const=0, LogicOutDataTypeMode=uint8, ZeroCross=off}
      mask prompts: relop "Operator:"; const "Constant value:"; LogicOutDataTypeMode "Output data type mode:"; ZeroCross "Enable zero crossing detection"
      mask help: Determine how a signal compares to a constant.
      mask init: same as HQEV_MiL_20160830_integrate_r2017a/MiL/Test_Integration/Driver/Driver/Driver_AutoPedal/CTRL AccPed/Brake off
      mask TypeOptions relop: == | ~= | < | <= | >= | >
      mask TypeOptions LogicOutDataTypeMode: uint8 | boolean
      mask Callback ZeroCross: sl('zeroCrossEnable', gcbh);
      mask Display: disp(str)
  Compare To Constant7 : Subsystem  mask(Compare To Constant){relop===, const=0, LogicOutDataTypeMode=uint8, ZeroCross=off}
      mask prompts: relop "Operator:"; const "Constant value:"; LogicOutDataTypeMode "Output data type mode:"; ZeroCross "Enable zero crossing detection"
      mask help: Determine how a signal compares to a constant.
      mask init: same as HQEV_MiL_20160830_integrate_r2017a/MiL/Test_Integration/Driver/Driver/Driver_AutoPedal/CTRL AccPed/Brake off
      mask TypeOptions relop: == | ~= | < | <= | >= | >
      mask TypeOptions LogicOutDataTypeMode: uint8 | boolean
      mask Callback ZeroCross: sl('zeroCrossEnable', gcbh);
      mask Display: disp(str)
  Constant2 : Constant  Value=-0.5
  Logical Operator2 : Logic  Operator=OR  Inputs=3  AllPortsSameDT=off  OutDataTypeStr=boolean
  Logical Operator4 : Logic  AllPortsSameDT=off  OutDataTypeStr=boolean
  Logical Operator6 : Logic  Operator=NOT  Inputs=3  AllPortsSameDT=off  OutDataTypeStr=boolean
  Product1 : Product  RndMeth=Zero
  Relational Operator : RelationalOperator  Operator=<  OutDataTypeStr=boolean  RndMeth=Nearest
  Sign : Signum
  Brake_Reset : Outport
  wires:
  Compare To Constant7/1(y) -> Logical Operator4/1
  Logical Operator4/1 -> Logical Operator2/3
  Logical Operator6/1 -> Logical Operator4/2
  Compare To Constant2/1(y) -> Logical Operator2/1
  Sign/1 -> Product1/1
  Constant2/1 -> Product1/2
  Product1/1 -> Relational Operator/2
  Relational Operator/1 -> Logical Operator2/2
  v_error/1 -> Relational Operator/1
  v_Veh/1 -> Sign/1
  delta_v_set/1 -> Compare To Constant2/1(u)
  Logical Operator2/1 -> Brake_Reset/1
  Brake/1 -> Compare To Constant7/1(u)
  Brake_Set/1 -> Logical Operator6/1

== system HQEV_MiL_20160830_integrate_r2017a/MiL/Test_Integration/Driver/Driver/Driver_AutoPedal/CTRL BrakePed/S-R Flip-Flop ==
  S : Inport
  R : Inport  Port=2
  Demux : Demux  Outputs=2
  Logic : CombinatorialLogic  TruthTable=[0 1;1 0;0 1;0 1;1 0;1 0;0 0;0 0]
  Memory : Memory  X0=initial_condition  InheritSampleTime=on
  Mux : Mux  Inputs=3
  Q : Outport  InitialOutput=0
  !Q : Outport  Port=2  InitialOutput=1
  wires:
  R/1 -> Mux/2
  S/1 -> Mux/1
  Demux/1 -> Memory/1, Q/1
  Demux/2 -> !Q/1
  Logic/1 -> Demux/1
  Mux/1 -> Logic/1
  Memory/1 -> Mux/3

== system HQEV_MiL_20160830_integrate_r2017a/MiL/Test_Integration/Driver/Driver/Driver_AutoPedal/CTRL BrakePed/Set_Block ==
  delta_v_set : Inport
  v_error : Inport  Port=2
  Compare To Constant1 : Subsystem  mask(Compare To Constant){relop=<, const=0, LogicOutDataTypeMode=boolean, ZeroCross=off}
      mask prompts: relop "Operator:"; const "Constant value:"; LogicOutDataTypeMode "Output data type mode:"; ZeroCross "Enable zero crossing detection"
      mask help: Determine how a signal compares to a constant.
      mask init: same as HQEV_MiL_20160830_integrate_r2017a/MiL/Test_Integration/Driver/Driver/Driver_AutoPedal/CTRL AccPed/Brake off
      mask TypeOptions relop: == | ~= | < | <= | >= | >
      mask TypeOptions LogicOutDataTypeMode: uint8 | boolean
      mask Callback ZeroCross: sl('zeroCrossEnable', gcbh);
      mask Display: disp(str)
  Compare To Constant3 : Subsystem  mask(Compare To Constant){relop=>, const=0.5, LogicOutDataTypeMode=boolean, ZeroCross=off}
      mask prompts: relop "Operator:"; const "Constant value:"; LogicOutDataTypeMode "Output data type mode:"; ZeroCross "Enable zero crossing detection"
      mask help: Determine how a signal compares to a constant.
      mask init: same as HQEV_MiL_20160830_integrate_r2017a/MiL/Test_Integration/Driver/Driver/Driver_AutoPedal/CTRL AccPed/Brake off
      mask TypeOptions relop: == | ~= | < | <= | >= | >
      mask TypeOptions LogicOutDataTypeMode: uint8 | boolean
      mask Callback ZeroCross: sl('zeroCrossEnable', gcbh);
      mask Display: disp(str)
  Compare To Constant5 : Subsystem  mask(Compare To Constant){relop===, const=0, LogicOutDataTypeMode=boolean, ZeroCross=off}
      mask prompts: relop "Operator:"; const "Constant value:"; LogicOutDataTypeMode "Output data type mode:"; ZeroCross "Enable zero crossing detection"
      mask help: Determine how a signal compares to a constant.
      mask init: same as HQEV_MiL_20160830_integrate_r2017a/MiL/Test_Integration/Driver/Driver/Driver_AutoPedal/CTRL AccPed/Brake off
      mask TypeOptions relop: == | ~= | < | <= | >= | >
      mask TypeOptions LogicOutDataTypeMode: uint8 | boolean
      mask Callback ZeroCross: sl('zeroCrossEnable', gcbh);
      mask Display: disp(str)
  Compare To Constant6 : Subsystem  mask(Compare To Constant){relop=>, const=2, LogicOutDataTypeMode=boolean, ZeroCross=off}
      mask prompts: relop "Operator:"; const "Constant value:"; LogicOutDataTypeMode "Output data type mode:"; ZeroCross "Enable zero crossing detection"
      mask help: Determine how a signal compares to a constant.
      mask init: same as HQEV_MiL_20160830_integrate_r2017a/MiL/Test_Integration/Driver/Driver/Driver_AutoPedal/CTRL AccPed/Brake off
      mask TypeOptions relop: == | ~= | < | <= | >= | >
      mask TypeOptions LogicOutDataTypeMode: uint8 | boolean
      mask Callback ZeroCross: sl('zeroCrossEnable', gcbh);
      mask Display: disp(str)
  Logical Operator1 : Logic  AllPortsSameDT=off  OutDataTypeStr=boolean
  Logical Operator3 : Logic  AllPortsSameDT=off  OutDataTypeStr=boolean
  Logical Operator5 : Logic  Operator=OR  AllPortsSameDT=off  OutDataTypeStr=boolean
  Brake_set : Outport
  wires:
  Compare To Constant1/1(y) -> Logical Operator1/1
  Compare To Constant3/1(y) -> Logical Operator1/2
  Compare To Constant5/1(y) -> Logical Operator3/1
  Compare To Constant6/1(y) -> Logical Operator3/2
  Logical Operator1/1 -> Logical Operator5/1
  Logical Operator3/1 -> Logical Operator5/2
  delta_v_set/1 -> Compare To Constant1/1(u), Compare To Constant5/1(u)
  v_error/1 -> Compare To Constant3/1(u), Compare To Constant6/1(u)
  Logical Operator5/1 -> Brake_set/1

== system HQEV_MiL_20160830_integrate_r2017a/MiL/Test_Integration/Driver/Driver/Driver_AutoPedal/CTRL BrakePed/velocoty ==
  v_set [km/h] : Inport
  v_Veh [km/h] : Inport  Port=2
  Run_Forward : Subsystem
  delta_v_set : Outport
  v_error : Outport  Port=2
  wires:
  v_set [km/h]/1 -> Run_Forward/1(v_set)
  v_Veh [km/h]/1 -> Run_Forward/2(v_Veh)
  Run_Forward/1(delta_v_set) -> delta_v_set/1  "delta_v_set"
  Run_Forward/2(error) -> v_error/1  "error"

== system HQEV_MiL_20160830_integrate_r2017a/MiL/Test_Integration/Driver/Driver/Driver_AutoPedal/Stop_Indicator/v_Set<0 ==
  u : Inport
  Compare : RelationalOperator  OutDataTypeStr=uint(8)  ZeroCross=off  RndMeth=Nearest  InputSameDT=on
  Constant : Constant  Value=const  OutDataTypeStr=Inherit: Inherit via back propagation
  y : Outport
  wires:
  u/1 -> Compare/1
  Constant/1 -> Compare/2
  Compare/1 -> y/1
